simulink model "MEKFsim"  (R2020b)
settings: Solver=FixedStepAuto  StartTime=0.0  StopTime=tsimulation  FixedStep=delta_t  RelTol=1e-3
values from neighbouring files (symbols this model uses):
  a = tiledlayout(3,1)    [MEKF_Monte_Carlo_Plot_data.m]    (also in UKF_Monte_Carlo_Plot_data.m; main_SDA.m = 6678)
  b_offset = sat.sensors.gyro_bias    [MEKF_Monte_Carlo_simulation.m]    (also in UKF_Monte_Carlo_simulation.m; main_SDA.m; main_SDA_v2.m)
  b_offset2 = -1e-2    (= -0.01)    [MEKF_Monte_Carlo_simulation.m]    (also in UKF_Monte_Carlo_simulation.m; main_SDA.m; main_SDA_v2.m = 0)
  day = 1    [main_SDA.m]
  e = 0.001    [main_SDA.m]
  hours = 0    [main_SDA.m]
  i = 51.6    [main_SDA.m]
  m = 12    [MEKF_Monte_Carlo_simulation.m]    (also in UKF_Monte_Carlo_simulation.m; main_SDA.m = 10; main_SDA_v2.m)
  minutes = 0    [main_SDA.m]
  month = 1    [main_SDA.m]
  nmax = 2    [MEKF_Monte_Carlo_simulation.m]    (also in UKF_Monte_Carlo_simulation.m; main_SDA.m; main_SDA_v2.m)
  nu = 0    [main_SDA.m]
  O = 300.5    [main_SDA.m]
  o = 0    [main_SDA.m]
  PSDbias = sat.sensors.gyro_bias^2*Ts    [MEKF_Monte_Carlo_simulation.m]    (also in UKF_Monte_Carlo_simulation.m; main_SDA.m; main_SDA_v2.m)
  PSDcss = sat.sensors.sun_coarse_sigma^2*Tss    [MEKF_Monte_Carlo_simulation.m]    (also in UKF_Monte_Carlo_simulation.m; main_SDA.m; main_SDA_v2.m)
  PSDfss = sat.sensors.sun_sigma^2*Tss    [MEKF_Monte_Carlo_simulation.m]    (also in UKF_Monte_Carlo_simulation.m; main_SDA.m; main_SDA_v2.m)
  PSDgyro = sat.sensors.gyro_sigma^2*Ts    [MEKF_Monte_Carlo_simulation.m]    (also in UKF_Monte_Carlo_simulation.m; main_SDA.m; main_SDA_v2.m)
  PSDmtm = sat.sensors.mag_sigma^2*Tss    [MEKF_Monte_Carlo_simulation.m]    (also in UKF_Monte_Carlo_simulation.m; main_SDA.m; main_SDA_v2.m)
  seconds = 0    [main_SDA.m]
  Ts = 1    [MEKF_Monte_Carlo_simulation.m]    (also in UKF_Monte_Carlo_simulation.m; main_SDA.m = 0.5; main_SDA_v2.m = 0.5)
  Tss = 1    [MEKF_Monte_Carlo_simulation.m]    (also in UKF_Monte_Carlo_simulation.m; main_SDA.m = 0.5; main_SDA_v2.m = 0.5)
  Use_IGRF = 0    [MEKF_Monte_Carlo_simulation.m]    (also in UKF_Monte_Carlo_simulation.m; main_SDA.m; main_SDA_v2.m)
  year = 2020    [main_SDA.m]
undefined symbols (not defined in the file or in its folder): deg, DipoleMod, km, rad, s
libraries: aerolibutil x10, aerolibconvert2 x8, vrlib x8, simulink x6, sharedtransform x2, aerolibcelestial x2, sharedutil x1, My_library x1, aerolibgravity2 x1, DipoleModel x1, aerolibobsolete x1
settings Model: Creator=Ricardo  LastModifiedBy=colpari

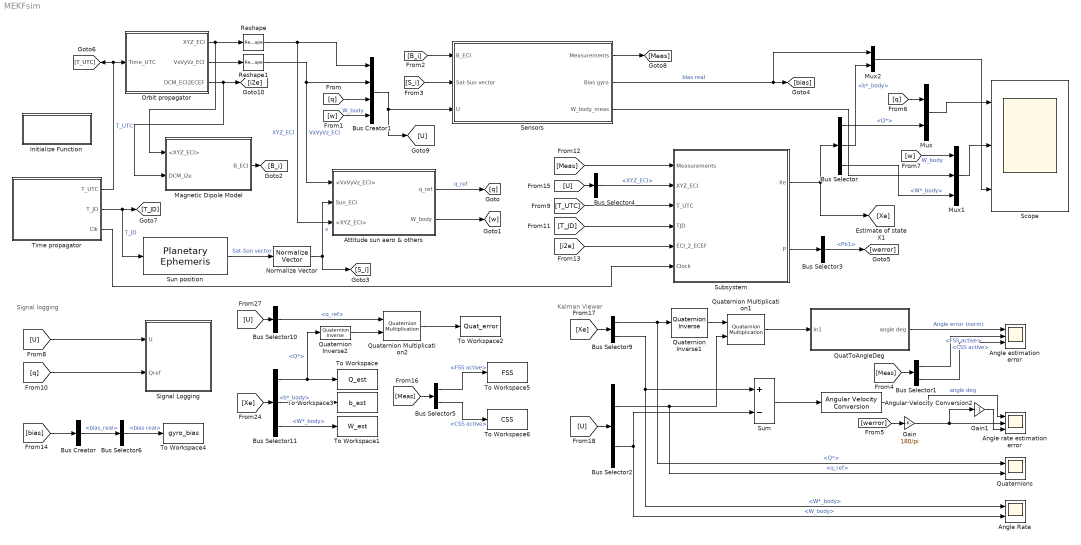
== system MEKFsim ==
  note: Signal logging
  note: Kalman Viewer
  Angle Rate : Scope  NumInputPorts=2
  Angle estimation error : Scope  NumInputPorts=3
  Angle rate estimation error : Scope  NumInputPorts=3
  Angular Velocity Conversion2 : aerolibconvert2/Angular Velocity Conversion  IU=rad/s  OU=deg/s
  Attitude sun aero & others : Subsystem
  Bus Creator : BusCreator  Inputs=1
  Bus Creator1 : BusCreator  Inputs=4
  Bus Selector : BusSelector  OutputSignals=Q*,b*_body,W*_body
  Bus Selector1 : BusSelector  OutputSignals=FSS active,CSS active
  Bus Selector10 : BusSelector  OutputSignals=q_ref
  Bus Selector11 : BusSelector  OutputSignals=Q*,b*_body,W*_body
  Bus Selector2 : BusSelector  OutputSignals=q_ref,W_body
  Bus Selector3 : BusSelector  OutputSignals=Pb1
  Bus Selector4 : BusSelector  OutputSignals=XYZ_ECI
  Bus Selector5 : BusSelector  OutputSignals=FSS active,CSS active
  Bus Selector6 : BusSelector  OutputSignals=bias real
  Bus Selector9 : BusSelector  OutputSignals=Q*,W*_body
  Gain : Gain  Gain=180/pi
  Gain1 : Gain  Gain=-1
  Initialize Function : Subsystem  TreatAsAtomicUnit=on
  Magnetic Dipole Model : Subsystem
  Mux : Mux  Inputs=2
  Mux1 : Mux  Inputs=3
  Mux2 : Mux  Inputs=2
  Normalize Vector : vrlib/Utilities/Normalize Vector  maxzero=0
  Orbit propagator : Subsystem
  QuatToAngleDeg : Subsystem
  Quaternion Inverse1 : aerolibutil/Quaternion Inverse
  Quaternion Inverse2 : aerolibutil/Quaternion Inverse
  Quaternion Multiplication1 : aerolibutil/Quaternion Multiplication
  Quaternion Multiplication2 : aerolibutil/Quaternion Multiplication
  Quaternions : Scope  NumInputPorts=2
  Reshape : Reshape
  Reshape1 : Reshape
  Scope : Scope  NumInputPorts=3
  Sensors : Subsystem
  Signal Logging : Subsystem
  Subsystem : Subsystem
  Sum : Sum  Inputs=+-
  Sun position : aerolibcelestial/Planetary Ephemeris  kmflag=km,km/s  epochflag=Julian date  de=DE405  nCenter=Earth  nTarget=Sun  errorflag=Error  velflag=off
      settings: SourceProductBaseCode=AE
  Time propagator : Subsystem
  To Workspace : ToWorkspace  VariableName=Q_est  SaveFormat=Timeseries  SampleTime=-1
  To Workspace1 : ToWorkspace  VariableName=W_est  SaveFormat=Timeseries  SampleTime=-1
  To Workspace2 : ToWorkspace  VariableName=Quat_error  SaveFormat=Timeseries  SampleTime=-1
  To Workspace3 : ToWorkspace  VariableName=b_est  SaveFormat=Timeseries  SampleTime=-1
  To Workspace4 : ToWorkspace  VariableName=gyro_bias  SaveFormat=Timeseries  SampleTime=-1
      settings: Save2DSignal=2-D array (concatenate along first dimension)
  To Workspace5 : ToWorkspace  VariableName=FSS  SaveFormat=Timeseries  SampleTime=-1
  To Workspace6 : ToWorkspace  VariableName=CSS  SaveFormat=Timeseries  SampleTime=-1
  wires:
  Orbit propagator/2(VxVyVz_ECI) -> Reshape1/1
  Orbit propagator/1(XYZ_ECI) -> Magnetic Dipole Model/1("<XYZ_ECI> "), Reshape/1
  Normalize Vector/1 -> [S_i], Attitude sun aero & others/2(Sun_ECI)  "x"
  Sun position/1 -> Normalize Vector/1  "Sat-Sun vector"
  Time propagator/1(T_UTC) -> [T_UTC], Orbit propagator/1("Time_UTC ")  "T_UTC"
  Attitude sun aero & others/1(q_ref) -> [q]  "q_ref"
  Time propagator/2(T_JD) -> Sun position/1, [T_JD]  "T_JD"
  Orbit propagator/3(DCM_ECI2ECEF) -> [i2e], Magnetic Dipole Model/2("DCM_i2e ")
  Magnetic Dipole Model/1("B_ECI ") -> [B_i]
  Attitude sun aero & others/2(W_body) -> [w]
  [q] -> Bus Creator1/3
  [w] -> Bus Creator1/4  "W_body"
  Bus Creator1/1 -> [U], Sensors/3(U)
  [B_i] -> Sensors/1(B_ECI)
  [S_i] -> Sensors/2(Sat-Sun vector)
  [q] -> Mux/1
  Bus Selector/1 -> Mux/2  "<Q*>"
  Bus Selector/3 -> Mux1/3  "<W*_body>"
  [w] -> Mux1/1  "W_body"
  Sensors/3(W_body_meas) -> Mux1/2
  Mux/1 -> Scope/1
  Mux1/1 -> Scope/2
  Bus Selector11/1 -> Quaternion Inverse2/1, To Workspace/1  "<Q*>"
  Bus Selector10/1 -> Quaternion Multiplication2/1  "<q_ref>"
  [q] -> Signal Logging/2(Qref)
  Quaternion Inverse2/1 -> Quaternion Multiplication2/2
  Quaternion Multiplication2/1 -> To Workspace2/1
  [U] -> Bus Selector10/1
  [Xe] -> Bus Selector11/1
  [U] -> Signal Logging/1(U)
  Bus Selector11/3 -> To Workspace1/1  "<W*_body>"
  Quaternion Multiplication1/1 -> QuatToAngleDeg/1(In1)
  Bus Selector1/2 -> Angle estimation error/3  "<CSS active>"
  QuatToAngleDeg/1(angle deg) -> Angle estimation error/1  "Angle error (norm)"
  Angular Velocity Conversion2/1 -> Angle rate estimation error/1  "angle deg"
  Bus Selector2/1 -> Quaternions/2, Quaternion Multiplication1/2  "<q_ref>"
  Bus Selector1/1 -> Angle estimation error/2  "<FSS active>"
  Bus Selector2/2 -> Sum/2, Angle Rate/2  "<W_body>"
  Sum/1 -> Angular Velocity Conversion2/1
  [Xe] -> Bus Selector9/1
  Bus Selector9/1 -> Quaternions/1, Quaternion Inverse1/1  "<Q*>"
  Bus Selector9/2 -> Angle Rate/1, Sum/1  "<W*_body>"
  Quaternion Inverse1/1 -> Quaternion Multiplication1/1
  [U] -> Bus Selector2/1
  [T_UTC] -> Subsystem/3(T_UTC)
  [T_JD] -> Subsystem/4(TJD)
  Bus Selector4/1 -> Subsystem/2(XYZ_ECI)  "<XYZ_ECI>"
  [U] -> Bus Selector4/1
  Subsystem/1(Xe) -> [Xe], Bus Selector/1
  Subsystem/2(P) -> Bus Selector3/1
  Gain1/1 -> Angle rate estimation error/3
  Bus Selector3/1 -> [werror]  "<Pb1>"
  [werror] -> Gain/1
  Gain/1 -> Gain1/1, Angle rate estimation error/2
  Reshape1/1 -> Bus Creator1/2, Attitude sun aero & others/1(<VxVyVz_ECI>)  "VxVyVz_ECI"
  Reshape/1 -> Attitude sun aero & others/3(<XYZ_ECI>), Bus Creator1/1  "XYZ_ECI"
  [i2e] -> Subsystem/5(ECI_2_ECEF)
  Time propagator/3(Clk) -> Subsystem/6(Clock)
  Sensors/2(Bias gyro) -> [bias], Mux2/1  "bias real"
  Bus Selector/2 -> Mux2/2  "<b*_body>"
  Mux2/1 -> Scope/3
  Sensors/1(Measurements) -> [Meas]
  [Meas] -> Subsystem/1(Measurements)
  [Meas] -> Bus Selector1/1
  Bus Selector11/2 -> To Workspace3/1  "<b*_body>"
  [bias] -> Bus Creator/1
  Bus Selector5/1 -> To Workspace5/1  "<FSS active>"
  [Meas] -> Bus Selector5/1
  Bus Selector5/2 -> To Workspace6/1  "<CSS active>"
  Bus Creator/1 -> Bus Selector6/1  "<bias_real>"
  Bus Selector6/1 -> To Workspace4/1  "<bias real>"

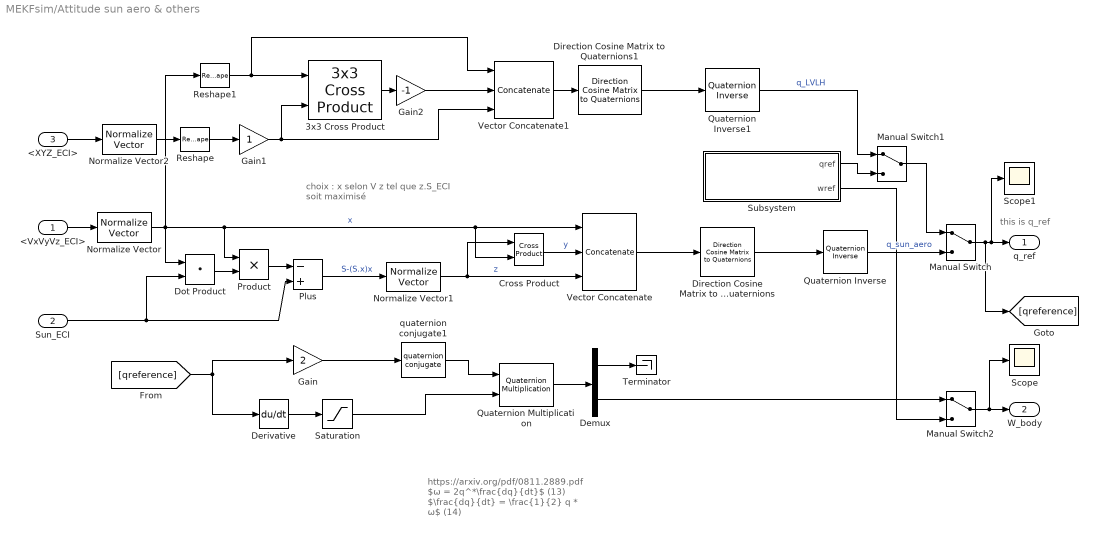
== system MEKFsim/Attitude sun aero & others ==
  note: this is q_ref
  note: choix :
      | x selon V
      | z tel que z.S_ECI soit maximisé
  note: https://arxiv.org/pdf/0811.2889.pdf
      | $ω = 2q^*\frac{dq}{dt}$ (13)
      |
      | $\frac{dq}{dt} = \frac{1}{2} q * ω$ (14)
  <VxVyVz_ECI> : Inport
  Sun_ECI : Inport  Port=2
  <XYZ_ECI> : Inport  Port=3
  3x3 Cross Product : sharedutil/3x3 Cross Product  aMode=aMode
      settings: SourceProductBaseCode=AE,PW,MT,UV,VE,VP
  Cross Product : vrlib/Utilities/Cross Product
  Demux : Demux  Outputs=[1 3]
  Derivative : Derivative
  Direction Cosine Matrix to Quaternions : sharedtransform/Direction Cosine Matrix  to Quaternions  aMode=0  action=None  tolerance=eps(2)
      settings: SourceProductBaseCode=AE,PW,MT,UV,VE,VP
  Direction Cosine Matrix to Quaternions1 : sharedtransform/Direction Cosine Matrix  to Quaternions  aMode=0  action=None  tolerance=eps(2)
      settings: SourceProductBaseCode=AE,PW,MT,UV,VE,VP
  Dot Product : DotProduct  InputSameDT=on  OutDataTypeStr=Inherit: Inherit via internal rule
  Gain : Gain  Gain=2
  Gain1 : Gain
  Gain2 : Gain  Gain=-1
  Manual Switch : ManualSwitch
  Manual Switch1 : ManualSwitch
  Manual Switch2 : ManualSwitch
  Normalize Vector : vrlib/Utilities/Normalize Vector  maxzero=0
  Normalize Vector1 : vrlib/Utilities/Normalize Vector  maxzero=0
  Normalize Vector2 : vrlib/Utilities/Normalize Vector  maxzero=0
  Plus : Sum  Inputs=-+
  Product : Product
  Quaternion Inverse : aerolibutil/Quaternion Inverse
  Quaternion Inverse1 : aerolibutil/Quaternion Inverse
  Quaternion Multiplication : aerolibutil/Quaternion Multiplication
  Reshape : Reshape  OutputDimensionality=Column vector (2-D)
  Reshape1 : Reshape  OutputDimensionality=Column vector (2-D)
  Saturation : Saturate  UpperLimit=5.5e-4  LowerLimit=-5.5e-4
  Scope : Scope
  Scope1 : Scope
  Subsystem : Subsystem
  Terminator : Terminator
  Vector Concatenate : Concatenate  NumInputs=3  Mode=Multidimensional array  ConcatenateDimension=2
  Vector Concatenate1 : Concatenate  NumInputs=3  Mode=Multidimensional array  ConcatenateDimension=2
  quaternion conjugate1 : My_library/quaternion conjugate
      settings: SourceProductName=My Library
  q_ref : Outport  VectorParamsAs1DForOutWhenUnconnected=off
  W_body : Outport  Port=2  VectorParamsAs1DForOutWhenUnconnected=off
  wires:
  Product/1 -> Plus/1
  Dot Product/1 -> Product/2
  Cross Product/1 -> Vector Concatenate/2  "y"
  Normalize Vector1/1 -> Vector Concatenate/3, Cross Product/1  "z"
  Plus/1 -> Normalize Vector1/1  "S-(S.x)x"
  Sun_ECI/1 -> Dot Product/2, Plus/2
  Vector Concatenate/1 -> Direction Cosine Matrix to Quaternions/1
  Direction Cosine Matrix to Quaternions/1 -> Quaternion Inverse/1
  Normalize Vector/1 -> Reshape1/1, Dot Product/1, Vector Concatenate/1, Cross Product/2, Product/1  "x"
  [qreference] -> Derivative/1, Gain/1
  Demux/1 -> Terminator/1
  Gain/1 -> quaternion conjugate1/1
  Demux/2 -> Manual Switch2/1
  Quaternion Multiplication/1 -> Demux/1
  quaternion conjugate1/1 -> Quaternion Multiplication/1
  Derivative/1 -> Saturation/1
  Manual Switch/1 -> [qreference], Scope1/1, q_ref/1
  Quaternion Inverse/1 -> Manual Switch/2  "q_sun_aero"
  3x3 Cross Product/1 -> Gain2/1
  Gain2/1 -> Vector Concatenate1/2
  Vector Concatenate1/1 -> Direction Cosine Matrix to Quaternions1/1
  Gain1/1 -> 3x3 Cross Product/2, Vector Concatenate1/3
  Normalize Vector2/1 -> Reshape/1
  Reshape/1 -> Gain1/1
  <XYZ_ECI>/1 -> Normalize Vector2/1
  Quaternion Inverse1/1 -> Manual Switch1/1  "q_LVLH"
  Direction Cosine Matrix to Quaternions1/1 -> Quaternion Inverse1/1
  <VxVyVz_ECI>/1 -> Normalize Vector/1
  Reshape1/1 -> 3x3 Cross Product/1, Vector Concatenate1/1
  Manual Switch1/1 -> Manual Switch/1
  Subsystem/1(qref) -> Manual Switch1/2
  Manual Switch2/1 -> Scope/1, W_body/1
  Subsystem/2(wref) -> Manual Switch2/2
  Saturation/1 -> Quaternion Multiplication/2

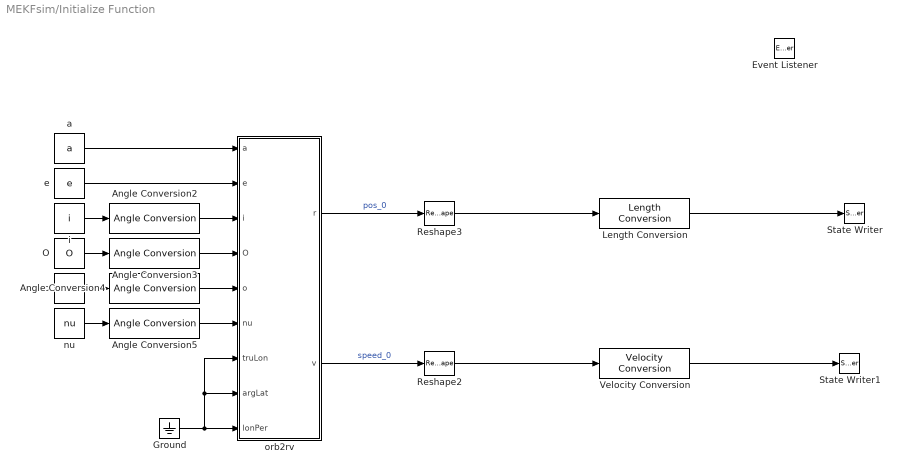
== system MEKFsim/Initialize Function ==
  Angle Conversion{2..5} (4 alike) : aerolibconvert2/Angle Conversion  IU=deg  OU=rad
  Event Listener : EventListener  DisableCoverage=on  EventName=reset
  Ground : Ground
  Length Conversion : aerolibconvert2/Length Conversion  IU=km  OU=m
  O : Constant  Value=O
  Reshape2 : Reshape  OutputDimensionality=Column vector (2-D)
  Reshape3 : Reshape  OutputDimensionality=Column vector (2-D)
  State Writer : StateWriter  StateOwnerBlock=../../Orbit propagator/Integrator_pos
  State Writer1 : StateWriter  StateOwnerBlock=../../Orbit propagator/Integrator_speed
  Velocity Conversion : aerolibconvert2/Velocity Conversion  IU=km/s  OU=m/s
  a : Constant  Value=a
  e : Constant  Value=e
  i : Constant  Value=i
  nu : Constant  Value=nu
  o : Constant  Value=o
  orb2rv : MATLAB Function  TreatAsAtomicUnit=on
  wires:
  Angle Conversion2/1 -> orb2rv/3(i)
  Length Conversion/1 -> State Writer/1
  Angle Conversion4/1 -> orb2rv/5(o)
  nu/1 -> Angle Conversion5/1
  Angle Conversion3/1 -> orb2rv/4(O)
  e/1 -> orb2rv/2(e)
  Reshape3/1 -> Length Conversion/1
  O/1 -> Angle Conversion3/1
  a/1 -> orb2rv/1(a)
  i/1 -> Angle Conversion2/1
  orb2rv/1(r) -> Reshape3/1  "pos_0"
  o/1 -> Angle Conversion4/1
  Angle Conversion5/1 -> orb2rv/6(nu)
  Velocity Conversion/1 -> State Writer1/1
  Reshape2/1 -> Velocity Conversion/1
  orb2rv/2(v) -> Reshape2/1  "speed_0"
  Ground/1 -> orb2rv/8(argLat), orb2rv/7(truLon), orb2rv/9(lonPer)

== system MEKFsim/Magnetic Dipole Model ==
  "<XYZ_ECI> " : Inport
  "DCM_i2e " : Inport  Port=2
  Bus Creator : BusCreator  Inputs=3
  ECEF To LLA : MATLAB Function  TreatAsAtomicUnit=on
  Interpreted MATLAB Function : MATLABFcn  MATLABFcn=DipoleMod(u(1),u(2),u(3),nmax)
  Permute Dimensions : PermuteDimensions
  Product : Product  Multiplication=Matrix(*)
  Product1 : Product  Multiplication=Matrix(*)
  Reshape : Reshape  OutputDimensionality=Row vector (2-D)
  scaling from nT to T : Gain  Gain=1e-9
  "B_ECI " : Outport  VectorParamsAs1DForOutWhenUnconnected=off
  wires:
  Reshape/1 -> Product/1
  Product/1 -> ECEF To LLA/1(X_ECEF)
  "<XYZ_ECI> "/1 -> Reshape/1
  ECEF To LLA/1(h) -> Bus Creator/1
  ECEF To LLA/2(lat) -> Bus Creator/2
  ECEF To LLA/3(long) -> Bus Creator/3
  Bus Creator/1 -> Interpreted MATLAB Function/1
  Interpreted MATLAB Function/1 -> Product1/2
  scaling from nT to T/1 -> "B_ECI "/1
  "DCM_i2e "/1 -> Product/2, Permute Dimensions/1
  Permute Dimensions/1 -> Product1/1
  Product1/1 -> scaling from nT to T/1

== system MEKFsim/Orbit propagator ==
  "Time_UTC " : Inport
  1/m : Gain  Gain=1/m
  Integrator_pos : Integrator
  Integrator_speed : Integrator
  Reshape : Reshape  OutputDimensionality=Column vector (2-D)
  Reshape2 : Reshape  OutputDimensionality=Column vector (2-D)
  Spherical Harmonic Gravity : Subsystem  TreatAsAtomicUnit=on  SystemSampleTime=1
  m : Gain  Gain=m
  XYZ_ECI : Outport  VectorParamsAs1DForOutWhenUnconnected=off
  VxVyVz_ECI : Outport  Port=2
  DCM_ECI2ECEF : Outport  Port=3
  wires:
  Integrator_pos/1 -> Reshape2/1, XYZ_ECI/1  "XYZ_ECI"
  Integrator_speed/1 -> VxVyVz_ECI/1, Integrator_pos/1  "VxVyVz_ECI"
  1/m/1 -> Integrator_speed/1  "AxAyAz_ECI"
  Reshape/1 -> 1/m/1
  m/1 -> Reshape/1  "Force_ECI"
  Spherical Harmonic Gravity/1(g_ECI (m/s²)) -> m/1
  "Time_UTC "/1 -> Spherical Harmonic Gravity/2(Time_UTC)
  Reshape2/1 -> Spherical Harmonic Gravity/1(XYZ_ECI)
  Spherical Harmonic Gravity/2(DCM_ECI2ECEF) -> DCM_ECI2ECEF/1

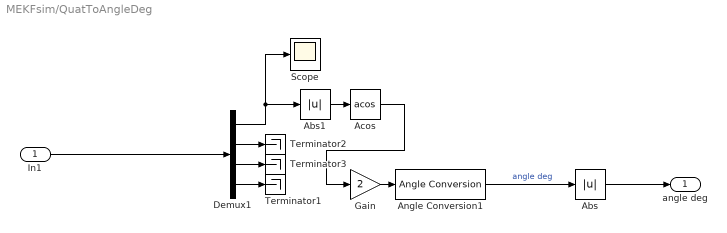
== system MEKFsim/QuatToAngleDeg ==
  In1 : Inport
  Abs : Abs
  Abs1 : Abs
  Acos : Trigonometry  Operator=acos
  Angle Conversion1 : aerolibconvert2/Angle Conversion  IU=rad  OU=deg
  Demux1 : Demux
  Gain : Gain  Gain=2
  Scope : Scope
  Terminator1 : Terminator
  Terminator2 : Terminator
  Terminator3 : Terminator
  angle deg : Outport  VectorParamsAs1DForOutWhenUnconnected=off
  wires:
  Acos/1 -> Gain/1
  Demux1/4 -> Terminator1/1
  In1/1 -> Demux1/1
  Angle Conversion1/1 -> Abs/1  "angle deg"
  Demux1/2 -> Terminator2/1
  Demux1/3 -> Terminator3/1
  Abs/1 -> angle deg/1
  Demux1/1 -> Abs1/1, Scope/1
  Gain/1 -> Angle Conversion1/1
  Abs1/1 -> Acos/1

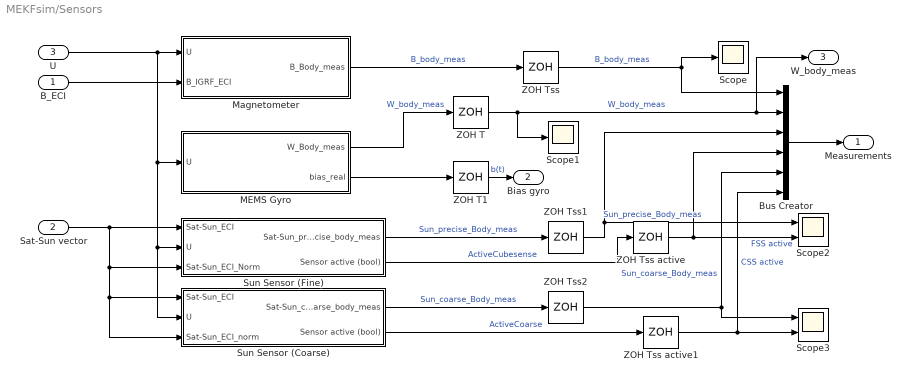
== system MEKFsim/Sensors ==
  B_ECI : Inport
  Sat-Sun vector : Inport  Port=2
  U : Inport  Port=3
  Bus Creator : BusCreator  Inputs=6
  MEMS Gyro : Subsystem
  Magnetometer : Subsystem
  Scope : Scope
  Scope1 : Scope
  Scope2 : Scope  NumInputPorts=2
  Scope3 : Scope  NumInputPorts=2
  Sun Sensor (Coarse) : Subsystem
  Sun Sensor (Fine) : Subsystem
  ZOH T : ZeroOrderHold  SampleTime=Ts
  ZOH T1 : ZeroOrderHold  SampleTime=Ts
  ZOH Tss : ZeroOrderHold  SampleTime=Tss
  ZOH Tss active : ZeroOrderHold  SampleTime=Tss
  ZOH Tss active1 : ZeroOrderHold  SampleTime=Tss
  ZOH Tss1 : ZeroOrderHold  SampleTime=Tss
  ZOH Tss2 : ZeroOrderHold  SampleTime=Tss
  Measurements : Outport  VectorParamsAs1DForOutWhenUnconnected=off
  Bias gyro : Outport  Port=2
  W_body_meas : Outport  Port=3
  wires:
  Sat-Sun vector/1 -> Sun Sensor (Fine)/3(Sat-Sun_ECI_Norm), Sun Sensor (Coarse)/3(Sat-Sun_ECI_norm), Sun Sensor (Coarse)/1(Sat-Sun_ECI), Sun Sensor (Fine)/1(Sat-Sun_ECI)
  MEMS Gyro/1(W_Body_meas) -> ZOH T/1  "W_body_meas"
  U/1 -> MEMS Gyro/1(U), Sun Sensor (Coarse)/2(U), Sun Sensor (Fine)/2(U), Magnetometer/1(U)
  Magnetometer/1(B_Body_meas) -> ZOH Tss/1  "B_body_meas"
  Sun Sensor (Coarse)/1(Sat-Sun_coarse_body_meas) -> ZOH Tss2/1  "Sun_coarse_Body_meas"
  Sun Sensor (Fine)/2(Sensor active (bool)) -> ZOH Tss active/1  "ActiveCubesense"
  Sun Sensor (Coarse)/2(Sensor active (bool)) -> ZOH Tss active1/1  "ActiveCoarse"
  B_ECI/1 -> Magnetometer/2(B_IGRF_ECI)
  Sun Sensor (Fine)/1(Sat-Sun_precise_body_meas) -> ZOH Tss1/1  "Sun_precise_Body_meas"
  ZOH Tss/1 -> Bus Creator/1, Scope/1  "B_body_meas"
  ZOH T/1 -> Bus Creator/2, W_body_meas/1, Scope1/1  "W_body_meas"
  ZOH Tss1/1 -> Bus Creator/3, Scope2/1  "Sun_precise_Body_meas"
  ZOH Tss2/1 -> Bus Creator/5, Scope3/1  "Sun_coarse_Body_meas"
  MEMS Gyro/2(bias_real) -> ZOH T1/1
  ZOH T1/1 -> Bias gyro/1  "b(t)"
  ZOH Tss active1/1 -> Bus Creator/6, Scope3/2  "CSS active"
  ZOH Tss active/1 -> Bus Creator/4, Scope2/2  "FSS active"
  Bus Creator/1 -> Measurements/1

== system MEKFsim/Signal Logging ==
  U : Inport
  Qref : Inport  Port=2
  Bus Selector4 : BusSelector  OutputSignals=XYZ_ECI,VxVyVz_ECI,q_ref,W_body
  Reshape1 : Reshape
  Reshape3 : Reshape
  To Workspace : ToWorkspace  VariableName=sat_pos  SaveFormat=Timeseries  SampleTime=1
      settings: Save2DSignal=2-D array (concatenate along first dimension)
  To Workspace1 : ToWorkspace  VariableName=sat_speed  SaveFormat=Timeseries  SampleTime=1
      settings: Save2DSignal=2-D array (concatenate along first dimension)
  To Workspace2 : ToWorkspace  VariableName=sat_Q  SaveFormat=Timeseries  SampleTime=-1
      settings: Save2DSignal=2-D array (concatenate along first dimension)
  To Workspace3 : ToWorkspace  VariableName=sat_omega  SaveFormat=Timeseries  SampleTime=-1
      settings: Save2DSignal=2-D array (concatenate along first dimension)
  To Workspace5 : ToWorkspace  VariableName=sat_Qref  SaveFormat=Timeseries  SampleTime=-1
      settings: Save2DSignal=2-D array (concatenate along first dimension)
  wires:
  Bus Selector4/3 -> To Workspace2/1  "<q_ref>"
  Bus Selector4/4 -> Reshape3/1  "<W_body>"
  U/1 -> Bus Selector4/1
  Bus Selector4/2 -> To Workspace1/1  "<VxVyVz_ECI>"
  Bus Selector4/1 -> To Workspace/1  "<XYZ_ECI>"
  Qref/1 -> Reshape1/1
  Reshape1/1 -> To Workspace5/1
  Reshape3/1 -> To Workspace3/1

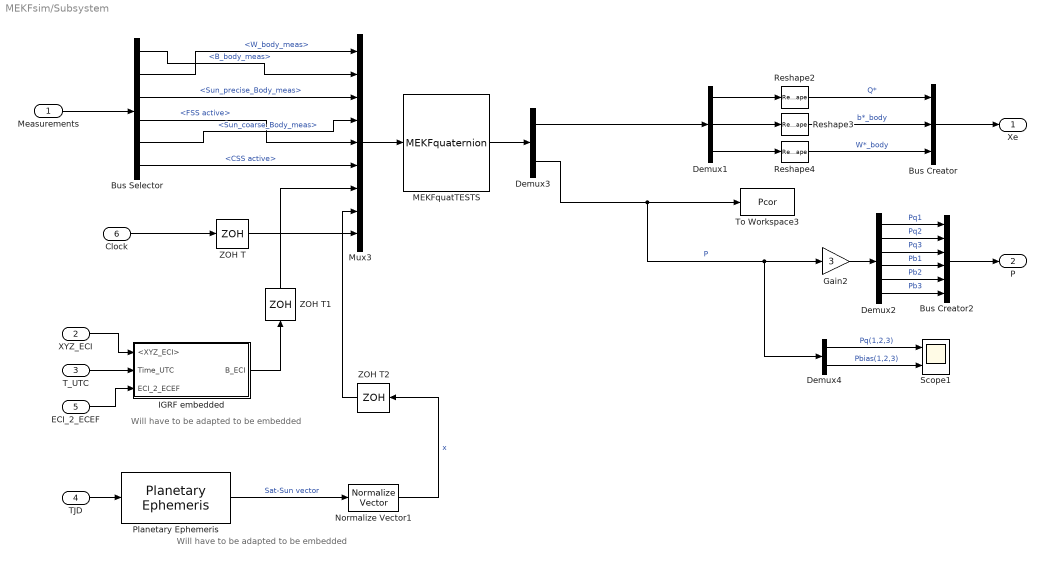
== system MEKFsim/Subsystem ==
  note: Will have to be adapted to be embedded
  note: Will have to be adapted to be embedded
  Measurements : Inport
  XYZ_ECI : Inport  Port=2
  T_UTC : Inport  Port=3
  TJD : Inport  Port=4
  ECI_2_ECEF : Inport  Port=5
  Clock : Inport  Port=6
  Bus Creator : BusCreator  Inputs=3
  Bus Creator2 : BusCreator  Inputs=6
  Bus Selector : BusSelector  OutputSignals=B_body_meas,W_body_meas,Sun_precise_Body_meas,FSS active,Sun_coarse_Body_meas,CSS active
  Demux1 : Demux  Outputs=3
  Demux2 : Demux  Outputs=6
  Demux3 : Demux  Outputs=[10;6]
  Demux4 : Demux  Outputs=[3 3]
  Gain2 : Gain  Gain=3
  IGRF embedded : Subsystem
  MEKFquatTESTS : MATLABFcn  MATLABFcn=MEKFquaternion
  Mux3 : Mux  Inputs=9
  Normalize Vector1 : vrlib/Utilities/Normalize Vector  maxzero=0
  Planetary Ephemeris : aerolibcelestial/Planetary Ephemeris  kmflag=km,km/s  epochflag=Julian date  de=DE405  nCenter=Earth  nTarget=Sun  errorflag=Error  velflag=off
      settings: SourceProductBaseCode=AE
  Reshape2 : Reshape  OutputDimensionality=Customize  OutputDimensions=[4]
  Reshape3 : Reshape  OutputDimensionality=Customize  OutputDimensions=[3]
  Reshape4 : Reshape  OutputDimensionality=Customize  OutputDimensions=[3]
  Scope1 : Scope  NumInputPorts=2
  To Workspace3 : ToWorkspace  VariableName=Pcor  SaveFormat=Timeseries  SampleTime=-1
  ZOH T : ZeroOrderHold  SampleTime=Ts
  ZOH T1 : ZeroOrderHold  SampleTime=Ts
  ZOH T2 : ZeroOrderHold  SampleTime=Ts
  Xe : Outport  VectorParamsAs1DForOutWhenUnconnected=off
  P : Outport  Port=2
  wires:
  Demux2/1 -> Bus Creator2/1  "Pq1"
  Bus Selector/6 -> Mux3/6  "<CSS active>"
  ZOH T/1 -> Mux3/9
  Measurements/1 -> Bus Selector/1
  ZOH T2/1 -> Mux3/8
  Bus Selector/5 -> Mux3/4  "<Sun_coarse_Body_meas>"
  Reshape3/1 -> Bus Creator/2  "b*_body"
  Gain2/1 -> Demux2/1
  Clock/1 -> ZOH T/1
  Demux4/1 -> Scope1/1  "Pq(1,2,3)"
  Demux4/2 -> Scope1/2  "Pbias(1,2,3)"
  Reshape4/1 -> Bus Creator/3  "W*_body"
  Mux3/1 -> MEKFquatTESTS/1
  TJD/1 -> Planetary Ephemeris/1
  ECI_2_ECEF/1 -> IGRF embedded/3(ECI_2_ECEF)
  Bus Creator2/1 -> P/1
  Demux2/4 -> Bus Creator2/4  "Pb1"
  Demux2/2 -> Bus Creator2/2  "Pq2"
  T_UTC/1 -> IGRF embedded/2("Time_UTC ")
  Demux2/6 -> Bus Creator2/6  "Pb3"
  Demux1/3 -> Reshape4/1
  Demux2/5 -> Bus Creator2/5  "Pb2"
  XYZ_ECI/1 -> IGRF embedded/1(<XYZ_ECI>)
  Demux3/2 -> Demux4/1, Gain2/1, To Workspace3/1  "P"
  Reshape2/1 -> Bus Creator/1  "Q*"
  Normalize Vector1/1 -> ZOH T2/1  "x"
  MEKFquatTESTS/1 -> Demux3/1
  Demux1/2 -> Reshape3/1
  Bus Selector/4 -> Mux3/5  "<FSS active>"
  ZOH T1/1 -> Mux3/7
  IGRF embedded/1(B_ECI) -> ZOH T1/1
  Demux1/1 -> Reshape2/1
  Planetary Ephemeris/1 -> Normalize Vector1/1  "Sat-Sun vector"
  Demux3/1 -> Demux1/1
  Demux2/3 -> Bus Creator2/3  "Pq3"
  Bus Creator/1 -> Xe/1
  Bus Selector/2 -> Mux3/1  "<W_body_meas>"
  Bus Selector/1 -> Mux3/2  "<B_body_meas>"
  Bus Selector/3 -> Mux3/3  "<Sun_precise_Body_meas>"

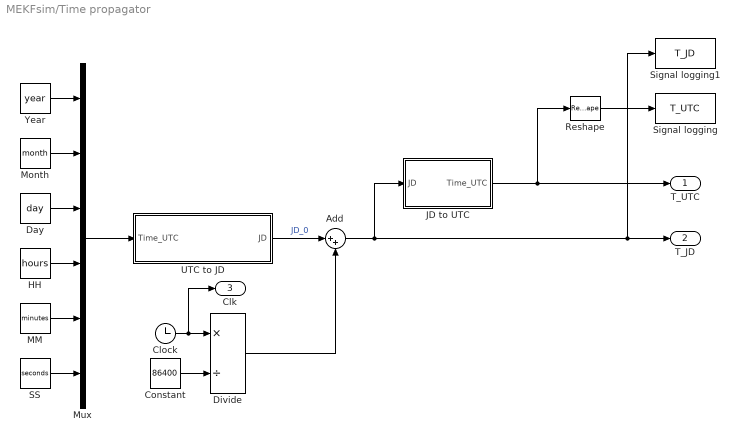
== system MEKFsim/Time propagator ==
  Add : Sum  Inputs=|++
  Clock : Clock
  Constant : Constant  Value=86400
  Day : Constant  Value=day
  Divide : Product  Inputs=*/
  HH : Constant  Value=hours
  JD to UTC : MATLAB Function  TreatAsAtomicUnit=on
  MM : Constant  Value=minutes
  Month : Constant  Value=month
  Mux : Mux  Inputs=6
  Reshape : Reshape
  SS : Constant  Value=seconds
  Signal logging : ToWorkspace  VariableName=T_UTC  SaveFormat=Timeseries  SampleTime=1
      settings: Save2DSignal=2-D array (concatenate along first dimension)
  Signal logging1 : ToWorkspace  VariableName=T_JD  SaveFormat=Timeseries  SampleTime=1
      settings: Save2DSignal=2-D array (concatenate along first dimension)
  UTC to JD : MATLAB Function  TreatAsAtomicUnit=on
  Year : Constant  Value=year
  T_UTC : Outport  VectorParamsAs1DForOutWhenUnconnected=off
  T_JD : Outport  Port=2  VectorParamsAs1DForOutWhenUnconnected=off
  Clk : Outport  Port=3
  wires:
  UTC to JD/1(JD) -> Add/1  "JD_0"
  Clock/1 -> Clk/1, Divide/1
  Constant/1 -> Divide/2
  JD to UTC/1(Time_UTC) -> T_UTC/1, Reshape/1
  Divide/1 -> Add/2
  Mux/1 -> UTC to JD/1(Time_UTC)
  Day/1 -> Mux/3
  Month/1 -> Mux/2
  Year/1 -> Mux/1
  HH/1 -> Mux/4
  MM/1 -> Mux/5
  SS/1 -> Mux/6
  Reshape/1 -> Signal logging/1
  Add/1 -> Signal logging1/1, T_JD/1, JD to UTC/1(JD)

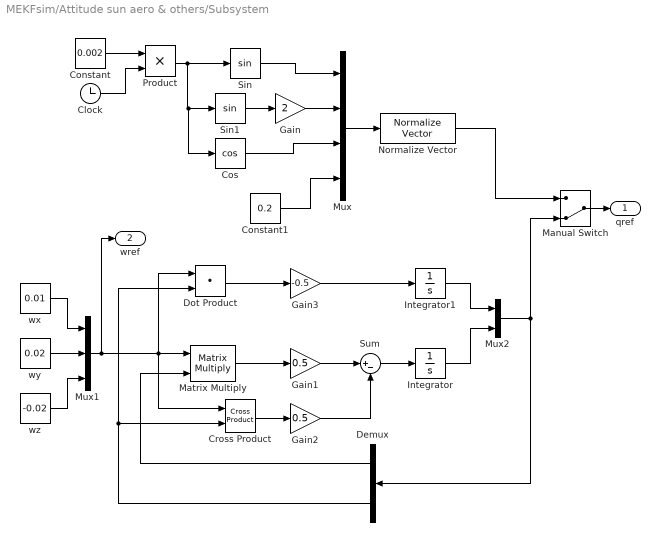
== system MEKFsim/Attitude sun aero & others/Subsystem ==
  Clock : Clock
  Constant : Constant  Value=0.002
  Constant1 : Constant  Value=0.2
  Cos : Trigonometry  Operator=cos
  Cross Product : vrlib/Utilities/Cross Product
  Demux : Demux  Outputs=[1;3]
  Dot Product : DotProduct  InputSameDT=on  OutDataTypeStr=Inherit: Inherit via internal rule
  Gain : Gain  Gain=2
  Gain1 : Gain  Gain=0.5
  Gain2 : Gain  Gain=0.5
  Gain3 : Gain  Gain=-0.5
  Integrator : Integrator  InitialCondition=[0;0;0]
  Integrator1 : Integrator  InitialCondition=1
  Manual Switch : ManualSwitch  CurrentSetting=0
  Matrix Multiply : Product  Multiplication=Matrix(*)
  Mux : Mux
  Mux1 : Mux  Inputs=3
  Mux2 : Mux  Inputs=[1;3]
  Normalize Vector : vrlib/Utilities/Normalize Vector  maxzero=0
  Product : Product
  Sin : Trigonometry
  Sin1 : Trigonometry
  Sum : Sum  Inputs=|+-
  wx : Constant  Value=0.01
  wy : Constant  Value=0.02
  wz : Constant  Value=-0.02
  qref : Outport
  wref : Outport  Port=2
  wires:
  Mux/1 -> Normalize Vector/1
  Normalize Vector/1 -> Manual Switch/1
  Constant/1 -> Product/1
  Clock/1 -> Product/2
  Product/1 -> Cos/1, Sin1/1, Sin/1
  Sin/1 -> Mux/1
  Sin1/1 -> Gain/1
  Gain/1 -> Mux/2
  Cos/1 -> Mux/3
  Constant1/1 -> Mux/4
  Manual Switch/1 -> qref/1
  wx/1 -> Mux1/1
  wy/1 -> Mux1/2
  wz/1 -> Mux1/3
  Mux1/1 -> wref/1, Dot Product/1, Cross Product/1, Matrix Multiply/1
  Matrix Multiply/1 -> Gain1/1
  Gain1/1 -> Sum/1
  Sum/1 -> Integrator/1
  Integrator/1 -> Mux2/2
  Mux2/1 -> Demux/1, Manual Switch/2
  Demux/1 -> Matrix Multiply/2
  Cross Product/1 -> Gain2/1
  Gain2/1 -> Sum/2
  Dot Product/1 -> Gain3/1
  Gain3/1 -> Integrator1/1
  Integrator1/1 -> Mux2/1
  Demux/2 -> Cross Product/2, Dot Product/2

== system MEKFsim/Orbit propagator/Spherical Harmonic Gravity ==
  note: Slower subsytem because it's too slow
  XYZ_ECI : Inport
  Time_UTC : Inport  Port=2
  ECI_2_ECEF : MATLABFcn  MATLABFcn=eci2ecef  OutputDimensions=[3,3]  Output1D=off
  Product : Product  Multiplication=Matrix(*)
  Product1 : Product  Inputs=/*  Multiplication=Matrix(*)
  Spherical Harmonic Gravity Model : aerolibgravity2/Spherical Harmonic Gravity Model  units=Metric (MKS)  degree=100  action=Warning  ptype=EGM2008  datafile='aerogmm2b.mat'
      settings: SourceProductBaseCode=AE
  Transpose : Math  Operator=transpose  SignedPower=on  SaturateOnIntegerOverflow=on
  g_ECI (m/s²) : Outport
  DCM_ECI2ECEF : Outport  Port=2
  wires:
  ECI_2_ECEF/1 -> DCM_ECI2ECEF/1, Product1/1, Product/1
  Transpose/1 -> Product1/2
  Product/1 -> Spherical Harmonic Gravity Model/1
  Spherical Harmonic Gravity Model/1 -> Transpose/1
  XYZ_ECI/1 -> Product/2
  Product1/1 -> g_ECI (m/s²)/1
  Time_UTC/1 -> ECI_2_ECEF/1

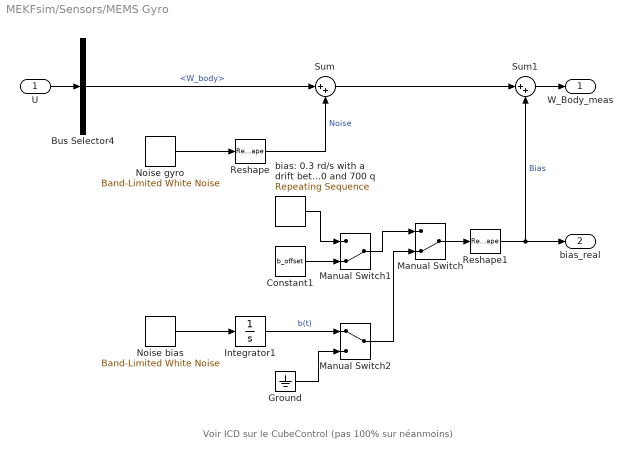
== system MEKFsim/Sensors/MEMS Gyro ==
  note: Voir ICD sur le CubeControl (pas 100% sur néanmoins)
  U : Inport
  Bus Selector4 : BusSelector  OutputSignals=W_body
  Constant1 : Constant  Value=b_offset
  Ground : Ground
  Integrator1 : Integrator  InitialCondition=b_offset
  Manual Switch : ManualSwitch  CurrentSetting=0
  Manual Switch1 : ManualSwitch  CurrentSetting=0
  Manual Switch2 : ManualSwitch
  Noise bias : simulink/Sources/Band-Limited White Noise  Cov=[PSDbias PSDbias PSDbias]  Ts=Ts  seed=[33341 95735 58375]
  Noise gyro : simulink/Sources/Band-Limited White Noise  Cov=[PSDgyro PSDgyro PSDgyro]  Ts=Ts  seed=[23341 48265 10583]
  Reshape : Reshape  OutputDimensionality=Column vector (2-D)
  Reshape1 : Reshape  OutputDimensionality=Column vector (2-D)
  Sum : Sum  Inputs=|++
  Sum1 : Sum  Inputs=|++
  bias: 0.3 rd/s with a drift between 400 and 700 q : simulink/Sources/Repeating Sequence  rep_seq_t="[0   400    700      1000]"  rep_seq_y=[b_offset b_offset b_offset+b_offset2 b_offset+b_offset2 ]
  W_Body_meas : Outport  VectorParamsAs1DForOutWhenUnconnected=off
  bias_real : Outport  Port=2
  wires:
  U/1 -> Bus Selector4/1
  Noise gyro/1 -> Reshape/1
  Sum/1 -> Sum1/1
  Reshape/1 -> Sum/2  "Noise"
  Bus Selector4/1 -> Sum/1  "<W_body>"
  Sum1/1 -> W_Body_meas/1
  Reshape1/1 -> bias_real/1, Sum1/2  "Bias"
  Manual Switch/1 -> Reshape1/1
  Manual Switch1/1 -> Manual Switch/1
  Constant1/1 -> Manual Switch1/2
  Noise bias/1 -> Integrator1/1
  bias: 0.3 rd/s with a drift between 400 and 700 q/1 -> Manual Switch1/1
  Integrator1/1 -> Manual Switch2/1  "b(t)"
  Ground/1 -> Manual Switch2/2
  Manual Switch2/1 -> Manual Switch/2

== system MEKFsim/Sensors/Magnetometer ==
  note: Valeur constructeur : 1-sigma = 50nT
  U : Inport
  B_IGRF_ECI : Inport  Port=2
  Bus Selector : BusSelector  OutputSignals=q_ref
  Noise MTM : simulink/Sources/Band-Limited White Noise  Cov=[PSDmtm PSDmtm PSDmtm]  Ts=Ts  seed=[23341 35825 59275]
  Quaternion Rotation : aerolibutil/Quaternion Rotation
  Reshape : Reshape  OutputDimensionality=Column vector (2-D)
  Sum : Sum  Inputs=|++
  B_Body_meas : Outport  VectorParamsAs1DForOutWhenUnconnected=off
  wires:
  B_IGRF_ECI/1 -> Quaternion Rotation/2
  Noise MTM/1 -> Reshape/1
  Quaternion Rotation/1 -> Sum/1  "B_IGRF_body"
  Sum/1 -> B_Body_meas/1
  Reshape/1 -> Sum/2
  U/1 -> Bus Selector/1
  Bus Selector/1 -> Quaternion Rotation/1  "<q_ref>"

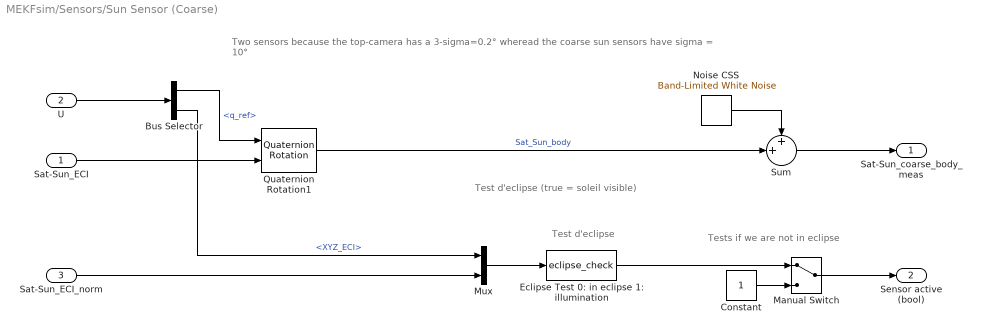
== system MEKFsim/Sensors/Sun Sensor (Coarse) ==
  note: Tests if we are not in eclipse
  note: Test d'eclipse (true = soleil visible)
  note: Two sensors because the top-camera has a 3-sigma=0.2° wheread the coarse sun sensors have sigma = 10°
  note: Test d'eclipse
  Sat-Sun_ECI : Inport
  U : Inport  Port=2
  Sat-Sun_ECI_norm : Inport  Port=3
  Bus Selector : BusSelector  OutputSignals=q_ref,XYZ_ECI
  Constant : Constant
  Eclipse Test 0: in eclipse 1: illumination : MATLABFcn  MATLABFcn=eclipse_check
  Manual Switch : ManualSwitch
  Mux : Mux  Inputs=2
  Noise CSS : simulink/Sources/Band-Limited White Noise  Cov=[PSDcss PSDcss PSDcss]  Ts=Tss  seed=[152 758 992]
  Quaternion Rotation1 : aerolibutil/Quaternion Rotation
  Sum : Sum  Inputs=++|
  Sat-Sun_coarse_body_meas : Outport  VectorParamsAs1DForOutWhenUnconnected=off
  Sensor active (bool) : Outport  Port=2  VectorParamsAs1DForOutWhenUnconnected=off
  wires:
  Sum/1 -> Sat-Sun_coarse_body_meas/1
  U/1 -> Bus Selector/1
  Sat-Sun_ECI/1 -> Quaternion Rotation1/2
  Bus Selector/1 -> Quaternion Rotation1/1  "<q_ref>"
  Quaternion Rotation1/1 -> Sum/2  "Sat_Sun_body"
  Eclipse Test 0: in eclipse 1: illumination/1 -> Manual Switch/1
  Mux/1 -> Eclipse Test 0: in eclipse 1: illumination/1
  Sat-Sun_ECI_norm/1 -> Mux/2
  Bus Selector/2 -> Mux/1  "<XYZ_ECI>"
  Constant/1 -> Manual Switch/2
  Manual Switch/1 -> Sensor active (bool)/1
  Noise CSS/1 -> Sum/1

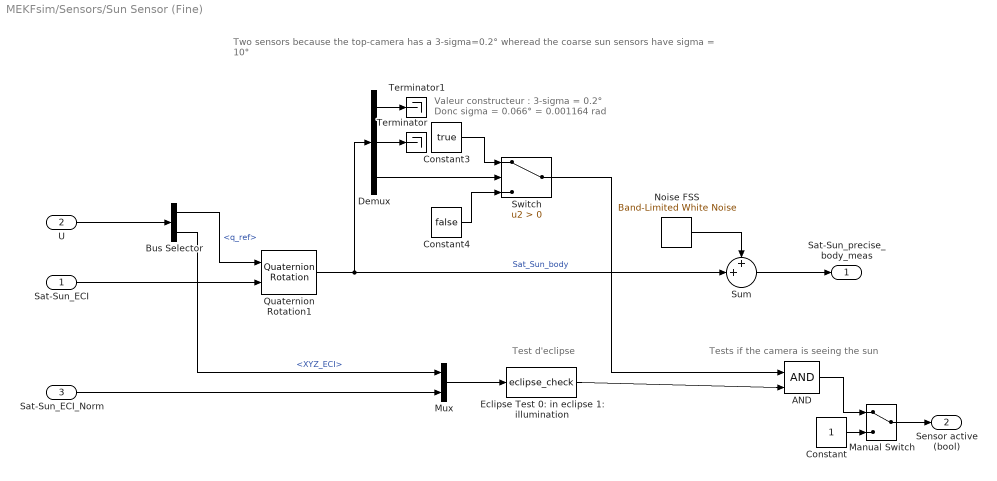
== system MEKFsim/Sensors/Sun Sensor (Fine) ==
  note: Tests if the camera is seeing the sun
  note: Test d'eclipse
  note: Two sensors because the top-camera has a 3-sigma=0.2° wheread the coarse sun sensors have sigma = 10°
  note: Valeur constructeur : 3-sigma = 0.2°
      | Donc sigma = 0.066° = 0.001164 rad
  Sat-Sun_ECI : Inport
  U : Inport  Port=2
  Sat-Sun_ECI_Norm : Inport  Port=3
  AND : Logic  IconShape=distinctive  AllPortsSameDT=off  OutDataTypeStr=boolean
  Bus Selector : BusSelector  OutputSignals=q_ref,XYZ_ECI
  Constant : Constant
  Constant3 : Constant  Value=true
  Constant4 : Constant  Value=false
  Demux : Demux  Outputs=3
  Eclipse Test 0: in eclipse 1: illumination : MATLABFcn  MATLABFcn=eclipse_check
  Manual Switch : ManualSwitch
  Mux : Mux  Inputs=2
  Noise FSS : simulink/Sources/Band-Limited White Noise  Cov=[PSDfss PSDfss PSDfss]  Ts=Tss  seed=[1 358 592]
  Quaternion Rotation1 : aerolibutil/Quaternion Rotation
  Sum : Sum  Inputs=++|
  Switch : Switch  Criteria=u2 > Threshold
  Terminator : Terminator
  Terminator1 : Terminator
  Sat-Sun_precise_body_meas : Outport  VectorParamsAs1DForOutWhenUnconnected=off
  Sensor active (bool) : Outport  Port=2  VectorParamsAs1DForOutWhenUnconnected=off
  wires:
  Switch/1 -> AND/1
  Sum/1 -> Sat-Sun_precise_body_meas/1
  U/1 -> Bus Selector/1
  Sat-Sun_ECI/1 -> Quaternion Rotation1/2
  Bus Selector/1 -> Quaternion Rotation1/1  "<q_ref>"
  Quaternion Rotation1/1 -> Sum/2, Demux/1  "Sat_Sun_body"
  Demux/3 -> Switch/2
  Constant3/1 -> Switch/1
  Demux/2 -> Terminator/1
  Demux/1 -> Terminator1/1
  Bus Selector/2 -> Mux/1  "<XYZ_ECI>"
  Eclipse Test 0: in eclipse 1: illumination/1 -> AND/2
  Constant4/1 -> Switch/3
  Mux/1 -> Eclipse Test 0: in eclipse 1: illumination/1
  Sat-Sun_ECI_Norm/1 -> Mux/2
  Constant/1 -> Manual Switch/2
  Manual Switch/1 -> Sensor active (bool)/1
  AND/1 -> Manual Switch/1
  Noise FSS/1 -> Sum/1

== system MEKFsim/Subsystem/IGRF embedded ==
  <XYZ_ECI> : Inport
  "Time_UTC " : Inport  Port=2
  ECI_2_ECEF : Inport  Port=3
  Bus Creator : BusCreator  Inputs=5
  Bus Selector4 : BusSelector  OutputSignals=XYZ_ECI
  Demux : Demux  Outputs=2
  ECI To LLA : MATLAB Function  TreatAsAtomicUnit=on
  Obtain B_ECI : Subsystem
  Product : Product  Multiplication=Matrix(*)
  Reshape : Reshape  OutputDimensionality=Row vector (2-D)
  Terminator : Terminator
  B_ECI : Outport  VectorParamsAs1DForOutWhenUnconnected=off
  wires:
  Demux/2 -> Terminator/1
  "Time_UTC "/1 -> Demux/1
  <XYZ_ECI>/1 -> Bus Selector4/1
  Reshape/1 -> Product/1
  Product/1 -> ECI To LLA/1(X_ECEF)
  Bus Selector4/1 -> Reshape/1  "<XYZ_ECI>"
  ECI To LLA/1(h) -> Bus Creator/1
  ECI To LLA/2(lat) -> Bus Creator/2
  ECI_2_ECEF/1 -> Bus Creator/5, Product/2  "DCM"
  ECI To LLA/3(long) -> Bus Creator/3
  Demux/1 -> Bus Creator/4
  Bus Creator/1 -> Obtain B_ECI/1(In1)
  Obtain B_ECI/1(Out1) -> B_ECI/1

== system MEKFsim/Subsystem/IGRF embedded/Obtain B_ECI ==
  In1 : Inport
  Dipole Subsystem : Subsystem  TreatAsAtomicUnit=on
  IGRF Subsystem : Subsystem  TreatAsAtomicUnit=on
  If : If
  Merge : Merge
  Use_IGRF : Constant  Value=Use_IGRF
  Out1 : Outport  VectorParamsAs1DForOutWhenUnconnected=off
  wires:
  If/1 -> IGRF Subsystem/Action
  In1/1 -> Dipole Subsystem/1(In1), IGRF Subsystem/1(In1)
  IGRF Subsystem/1(Out1) -> Merge/1
  Use_IGRF/1 -> If/1
  Merge/1 -> Out1/1
  Dipole Subsystem/1(Out1) -> Merge/2
  If/2 -> Dipole Subsystem/Action

== system MEKFsim/Subsystem/IGRF embedded/Obtain B_ECI/Dipole Subsystem ==
  In1 : Inport
  Action Port : ActionPort  ActionPortLabel=else
  Bus Selector1 : BusSelector  OutputSignals=h,lat,long,DCM
  Dipole Model : DipoleModel/Dipole Model  SystemSampleTime=-1  VariantActivationTime=update diagram  Latency=0  AutoFrameSizeCalculation=off
      link override Interpreted MATLAB Function: MATLABFcn=DipoleMod(u(1),u(2),u(3),nmaxKF)
  Out1 : Outport  VectorParamsAs1DForOutWhenUnconnected=off
  wires:
  In1/1 -> Bus Selector1/1
  Bus Selector1/3 -> Dipole Model/3  "<long>"
  Dipole Model/1 -> Out1/1
  Bus Selector1/1 -> Dipole Model/1  "<h>"
  Bus Selector1/2 -> Dipole Model/2  "<lat>"
  Bus Selector1/4 -> Dipole Model/4  "<DCM>"

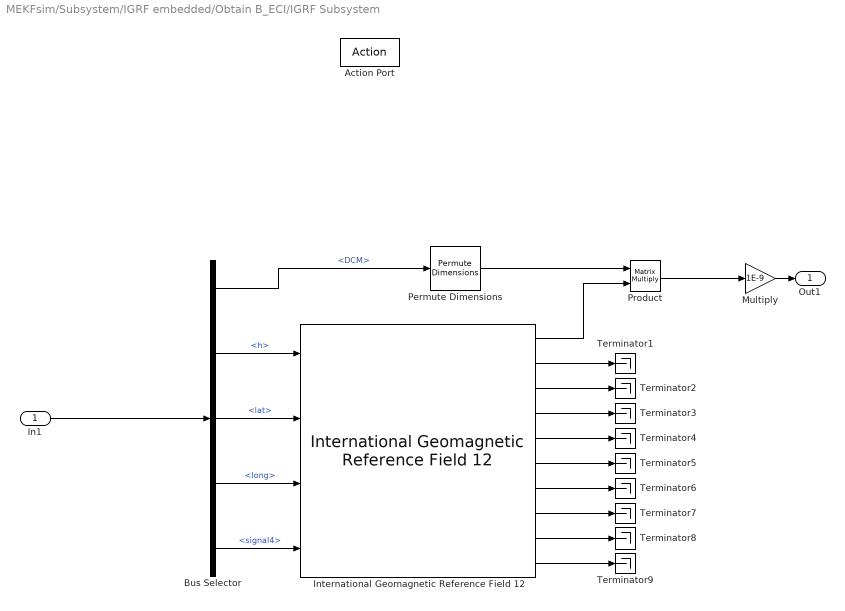
== system MEKFsim/Subsystem/IGRF embedded/Obtain B_ECI/IGRF Subsystem ==
  In1 : Inport
  Action Port : ActionPort  ActionPortLabel=if(u1 > 0)
  Bus Selector : BusSelector  OutputSignals=DCM,h,lat,long,signal4
  International Geomagnetic Reference Field 12 : aerolibobsolete/International Geomagnetic Reference Field 12  units=Metric (MKS)  time_in=on  month=January  day=1  year=2020  action=None  sv_out=on
      settings: SourceProductBaseCode=AE
  Multiply : Gain  Gain=1E-9
  Permute Dimensions : PermuteDimensions
  Product : Product  Multiplication=Matrix(*)
  Terminator{1..9} (9 alike) : Terminator
  Out1 : Outport  VectorParamsAs1DForOutWhenUnconnected=off
  wires:
  In1/1 -> Bus Selector/1
  Bus Selector/2 -> International Geomagnetic Reference Field 12/1  "<h>"
  Multiply/1 -> Out1/1
  Bus Selector/5 -> International Geomagnetic Reference Field 12/4  "<signal4>"
  Bus Selector/4 -> International Geomagnetic Reference Field 12/3  "<long>"
  Bus Selector/3 -> International Geomagnetic Reference Field 12/2  "<lat>"
  International Geomagnetic Reference Field 12/2 -> Terminator1/1
  International Geomagnetic Reference Field 12/10 -> Terminator9/1
  International Geomagnetic Reference Field 12/4 -> Terminator3/1
  International Geomagnetic Reference Field 12/5 -> Terminator4/1
  International Geomagnetic Reference Field 12/3 -> Terminator2/1
  International Geomagnetic Reference Field 12/1 -> Product/2
  International Geomagnetic Reference Field 12/6 -> Terminator5/1
  International Geomagnetic Reference Field 12/8 -> Terminator7/1
  International Geomagnetic Reference Field 12/7 -> Terminator6/1
  International Geomagnetic Reference Field 12/9 -> Terminator8/1
  Bus Selector/1 -> Permute Dimensions/1  "<DCM>"
  Permute Dimensions/1 -> Product/1
  Product/1 -> Multiply/1

== matlab function MEKFsim/Time propagator/JD to UTC ==
  data: JD input; Time_UTC output
function Time_UTC = fcn(JD)
    coder.extrinsic('datetime','datevec');
    Time_UTC = [0,0,0,0,0,0];
Time_UTC =  datevec(datetime(JD,'convertfrom','juliandate'));

== matlab function MEKFsim/Time propagator/UTC to JD ==
  data: Time_UTC input; JD output
function JD = fcn(Time_UTC)

% JD = juliandate(Time_UTC);
JD = Dt2jD(Time_UTC);

== matlab function MEKFsim/Subsystem/IGRF embedded/ECI To LLA ==
  data: X_ECEF input; h output; lat output; long output
function [h, lat, long] = fcn(X_ECEF)
    h = 0;
    lat = 0;
    long = 0;
[lat, long, h] = ecef2geod(X_ECEF(1),X_ECEF(2),X_ECEF(3));

== matlab function MEKFsim/Initialize Function/orb2rv ==
  data: a input; r output; e input; i input; O input; o input; nu input; v output; truLon input; argLat input; lonPer input
%----------------------- Begin Code Sequence -----------------------------%
% Purpose:                                                                %
% Convert a given set of Keplerian Orbital Elements to state vectors in   %
% in the ECI frame of reference                                           %
%                                                                         %
%-------------------------------------------------------------------------%
%                                                                         %
% Inputs:                                                                 %
%-------- 
%a                      [1 x N]                         Semimajor axis
%                                                       (km)
%
%e                      [1 x N]                         Eccentricity Magnitude
%                                                       (unitless)
%
%i                      [1 x N]                         inclination
%                                                       (radians)
%
%O                      [1 x N]                         Right Ascention of
%                                                       the ascending node
%                                                       (radians)
%
%o                      [1 x N]                         Argument of perigee
%                                                       (radians)
%
%nu                     [1 x N]                         True Anomaly
%                                                       (radians)
%
%truLon                 [1 x N]                         True Longitude
%                                                       (radians)
%
%argLat                 [1 x N]                         Argument of Latitude
%                                                       (radians)
%
%lonPer                 [1 x N]                         Longitude of Periapse
%                                                       (radians)
%
%mu                     double                          Gravitational Constant
%                                                       Defaults to Earth if
%                                                       not specified
%
% Outputs:
%---------                                                                %
%r_ECI                  [3 x N]                         Position Vector in
%                                                       ECI coordinate
%                                                       frame of reference
%
%v_ECI                  [3 x N]                         Velocity vector in
%                                                       ECI coordinate
%                                                       frame of reference
%
% References:
%-------------
%Vallado,D. Fundamentals of Astrodynamics and Applications. 2007.
%
% Function Dependencies:
%------------------
%None
%------------------------------------------------------------------       %
% Programed by Darin Koblick  03-04-2012                                  %
%------------------------------------------------------------------       %
function [r,v] = orb2rv(a,e,i,O,o,nu,truLon,argLat,lonPer)
mu = 398600.4418;
%Make all inputs consistent w/ dimensions
a = a(:); e = e(:); i = i(:); O = O(:); o = o(:); nu = nu(:);
if e<1
    p=a*(1-e*e);
else
    p=2*a;
end
ietol = 1e-8;
idx = e < ietol & mod(i,pi) < ietol;
if any(idx); o(idx) = 0; O(idx) = 0; nu(idx) = truLon(idx); end
idx = e < ietol & mod(i,pi) > ietol;
if any(idx); o(idx) = 0; nu(idx) = argLat(idx); end
idx = e > ietol & mod(i,pi) < ietol;
if any(idx); O(idx) = 0; o(idx) = lonPer(idx); end
%Find rPQW and vPQW
rPQW = cat(2,p.*cos(nu)./(1 +e.*cos(nu)),p.*sin(nu)./(1+e.*cos(nu)),zeros(size(nu)));
vPQW = cat(2,-sqrt(mu./p).*sin(nu),sqrt(mu./p).*(e+cos(nu)),zeros(size(nu)));
%Create Transformation Matrix
PQW2IJK = NaN(3,3,size(p,1));
cO = cos(O); sO = sin(O); co = cos(o); so = sin(o); ci = cos(i); si = sin(i);
PQW2IJK(1,1,:) = cO.*co-sO.*so.*ci; PQW2IJK(1,2,:) = -cO.*so-sO.*co.*ci; PQW2IJK(1,3,:) = sO.*si;
PQW2IJK(2,1,:) = sO.*co+cO.*so.*ci; PQW2IJK(2,2,:) = -sO.*so+cO.*co.*ci; PQW2IJK(2,3,:) = -cO.*si;
PQW2IJK(3,1,:) = so.*si;            PQW2IJK(3,2,:) = co.*si;             PQW2IJK(3,3,:) = ci;
%Transform rPQW and vPQW to rECI and vECI
r = multiDimMatrixMultiply(PQW2IJK,rPQW)';  
v = multiDimMatrixMultiply(PQW2IJK,vPQW)';
end
function c = multiDimMatrixMultiply(a,b)
c = NaN(size(b));
c(:,1) = sum(bsxfun(@times,a(1,:,:),permute(b,[3 2 1])),2);
c(:,2) = sum(bsxfun(@times,a(2,:,:),permute(b,[3 2 1])),2);
c(:,3) = sum(bsxfun(@times,a(3,:,:),permute(b,[3 2 1])),2);
end

== matlab function MEKFsim/Magnetic Dipole Model/ECEF To LLA ==
  data: X_ECEF input; h output; lat output; long output
function [h, lat, long] = fcn(X_ECEF)
    h = 0;
    lat = 0;
    long = 0;
[lat, long, h] = ecef2geod(X_ECEF(1),X_ECEF(2),X_ECEF(3));
